simulink model "simulation_singlecontroller"  (R2017a)
settings: Solver=VariableStepAuto  StartTime=0.0  StopTime=10.0  RelTol=1e-3
values from neighbouring files (symbols this model uses):
  C2 = H_gain*H_notch*H_Lead*H_pd*H_I*H_LP    [simulation_singlecontroller.m]
  CFF = tf([1],[1])    [simulation_singlecontroller.m]
  H2 = H2_plant*sysdelay    [model_estimation.m]    (also in model_fitting.m; nestedloop_script.m; simulation_singlecontroller.m)
  SampleTime = 1/SampleRate    (= 0.00048828125)    [encoderTfEst.m]    (also in model_estimation.m; model_fitting.m; nestedloop_script.m; simulation_singlecontroller.m)
settings Model: Creator=marce  LastModifiedBy=marce

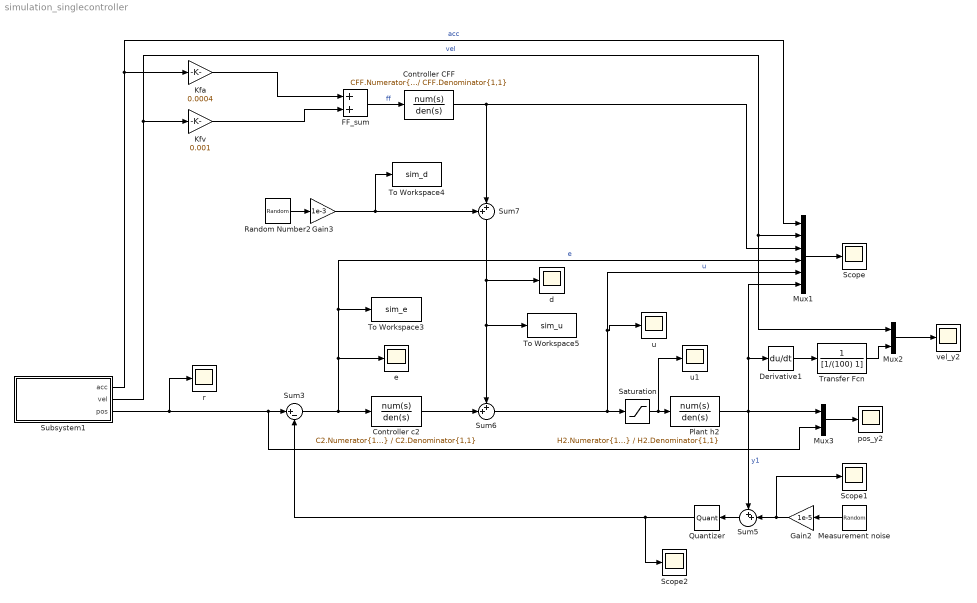
== system simulation_singlecontroller ==
  Controller CFF : TransferFcn  Numerator=CFF.Numerator{1,1}  Denominator=CFF.Denominator{1,1}
  Controller c2 : TransferFcn  Numerator=C2.Numerator{1,1}  Denominator=C2.Denominator{1,1}
  Derivative1 : Derivative
  "FF_sum " : Sum
  Gain2 : Gain  Gain=1e-5
  Gain3 : Gain  Gain=1e-3
  Kfa : Gain  Gain=0.0004
  Kfv : Gain  Gain=0.001
  Measurement noise : RandomNumber  Variance=2  SampleTime=SampleTime
  Mux1 : Mux  Inputs=6
  Mux2 : Mux  Inputs=2
  Mux3 : Mux  Inputs=2
  Plant h2 : TransferFcn  Numerator=H2.Numerator{1,1}  Denominator=H2.Denominator{1,1}
  Quantizer : Quantizer  QuantizationInterval=SampleTime
  Random Number2 : RandomNumber  SampleTime=SampleTime
  Saturation : Saturate  UpperLimit=2.5  LowerLimit=-2.5
  Scope : Scope
  Scope1 : Scope
  Scope2 : Scope
  Subsystem1 : Subsystem  mask(Ref3){}
      settings: OpenFcn=r3g_main
      mask Display: disp('Ref3');
  Sum3 : Sum  Inputs=|+-
  Sum5 : Sum  Inputs=++|
  Sum6 : Sum  Inputs=++|
  Sum7 : Sum  Inputs=++|
  To Workspace3 : ToWorkspace  VariableName=sim_e  SaveFormat=Timeseries  SampleTime=-1
  To Workspace4 : ToWorkspace  VariableName=sim_d  SaveFormat=Timeseries  SampleTime=-1
  To Workspace5 : ToWorkspace  VariableName=sim_u  SaveFormat=Timeseries  SampleTime=-1
  Transfer Fcn : TransferFcn  Denominator=[1/(100) 1]
  d : Scope
  e : Scope
  pos_y2 : Scope
  r : Scope
  u : Scope
  u1 : Scope
  vel_y2 : Scope
  wires:
  Kfa/1 -> "FF_sum "/1
  Kfv/1 -> "FF_sum "/2
  Subsystem1/1(acc) -> Mux1/1, Kfa/1  "acc"
  Mux1/1 -> Scope/1
  Saturation/1 -> u1/1, Plant h2/1
  Sum7/1 -> To Workspace5/1, Sum6/1, d/1
  Plant h2/1 -> Mux1/6, Derivative1/1, Mux3/1, Sum5/1  "y1"
  Sum3/1 -> e/1, Mux1/4, To Workspace3/1, Controller c2/1  "e"
  Random Number2/1 -> Gain3/1
  "FF_sum "/1 -> Controller CFF/1  "ff"
  Measurement noise/1 -> Gain2/1
  Subsystem1/3(pos) -> r/1, Mux3/2, Sum3/1
  Gain3/1 -> To Workspace4/1, Sum7/1
  Controller c2/1 -> Sum6/2
  Sum6/1 -> u/1, Mux1/5, Saturation/1  "u"
  Gain2/1 -> Sum5/2, Scope1/1
  Sum5/1 -> Quantizer/1
  Subsystem1/2(vel) -> Kfv/1, Mux2/1, Mux1/2  "vel"
  Controller CFF/1 -> Mux1/3, Sum7/2
  Mux3/1 -> pos_y2/1
  Transfer Fcn/1 -> Mux2/2
  Derivative1/1 -> Transfer Fcn/1
  Mux2/1 -> vel_y2/1
  Quantizer/1 -> Scope2/1, Sum3/2

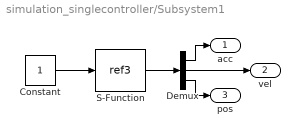
== system simulation_singlecontroller/Subsystem1 ==
  Constant : Constant
  Demux : Demux  Outputs=3
  S-Function : S-Function  FunctionName=ref3  Parameters=ref_part  SFunctionDeploymentMode=off  EnableBusSupport=off
      settings: OpenFcn=global ref_part; r3g_main
  acc : Outport
  vel : Outport  Port=2
  pos : Outport  Port=3
  wires:
  Constant/1 -> S-Function/1
  S-Function/1 -> Demux/1
  Demux/1 -> acc/1
  Demux/2 -> vel/1
  Demux/3 -> pos/1
